simulink model "Simulink_pid_temp_control"  (R2021a)
settings: Solver=VariableStepAuto  StartTime=0.0  StopTime=10.0  RelTol=1e-3
settings Model: Creator=Dell  LastModifiedBy=Dell

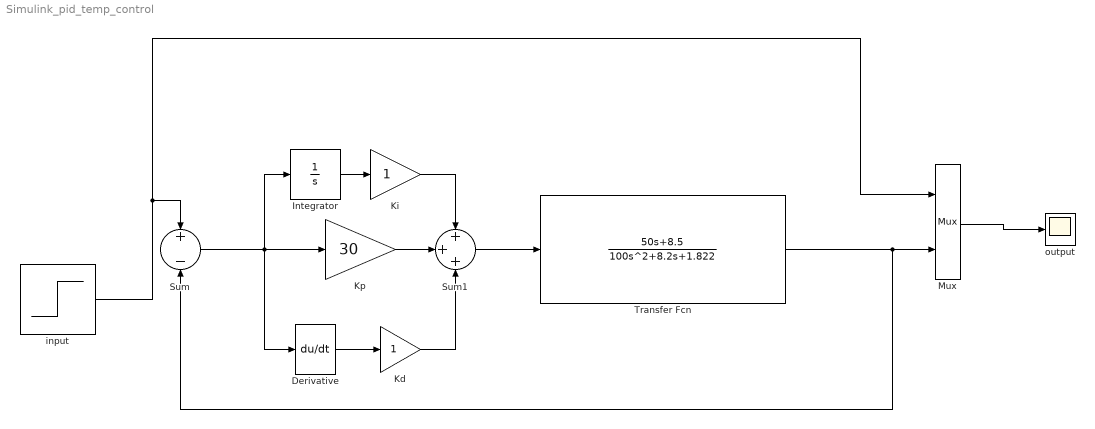
== system Simulink_pid_temp_control ==
  Derivative : Derivative
  Integrator : Integrator
  Kd : Gain
  Ki : Gain
  Kp : Gain  Gain=30
  Mux : Mux  Inputs=2
  Sum : Sum  Inputs=+-
  Sum1 : Sum  Inputs=+++
  Transfer Fcn : TransferFcn  Numerator=[50,8.5]  Denominator=[100,8.2,1.822]
  input : Step  SampleTime=0
  output : Scope
  wires:
  Kp/1 -> Sum1/2
  Ki/1 -> Sum1/1
  Sum/1 -> Derivative/1, Integrator/1, Kp/1
  input/1 -> Mux/1, Sum/1
  Derivative/1 -> Kd/1
  Sum1/1 -> Transfer Fcn/1
  Mux/1 -> output/1
  Transfer Fcn/1 -> Mux/2, Sum/2
  Kd/1 -> Sum1/3
  Integrator/1 -> Ki/1
